simulink model "power_PVarray_grid_det"  (Simulink 8.8)
settings: Solver=FixedStepDiscrete  StartTime=0.0  StopTime=14  RelTol=1e-3
PreLoadFcn:
  | Ts_Power=1e-6;
  | Ts_Control=100e-6;
undefined symbols (not defined in the file or in its folder): D1, Delta, DiscIntNeverNeededParam, sigbuilder_block
libraries: powerlib x23, powerlib_meascontrol x11, simulink x2, re_lib x1
(part 1 of 2)
Description:
  | Copyright 2008-2016 The MathWorks, Inc.
settings Model: SuppressorTable=22 serialization::archive 11 0 3 0 0 0 11 0  Creator=MathWorks  LastModifiedBy=oka  SimulationMode=accelerator
settings DataIOCC: SignalLogging=off  DSMLogging=off
settings OptimizationCC: ExpressionDepthLimit=2147483647
settings DebuggingCC: SolverPrmCheckMsg=warning
settings ConfigComp: CovSFcnEnable=off

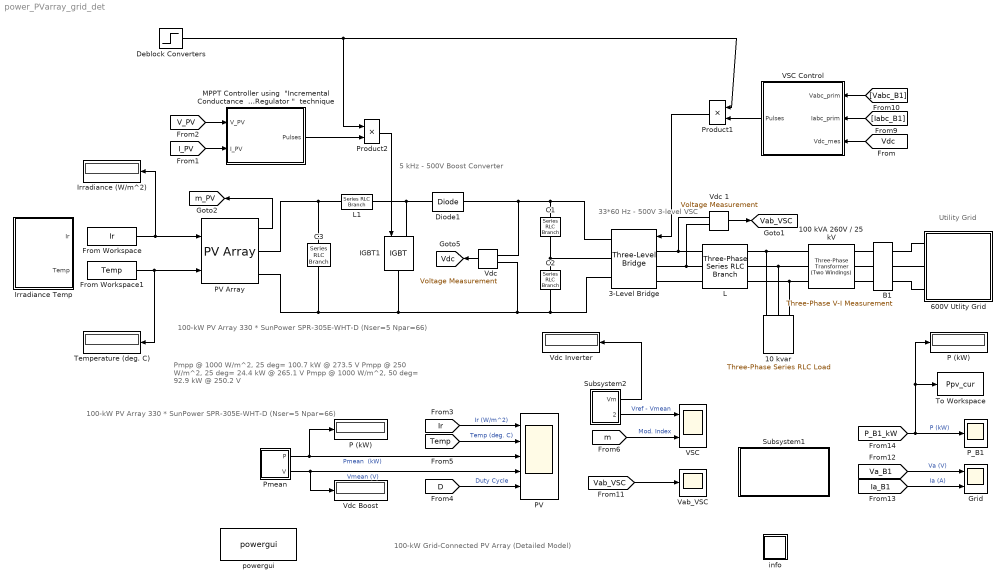
== system power_PVarray_grid_det ==
  note: 5 kHz - 500V
      | Boost Converter
  note: 33*60 Hz - 500V
      | 3-level VSC
  note: 100-kW Grid-Connected PV Array (Detailed Model)
  note: Utility Grid
  note: Pmpp @ 1000 W/m^2, 25 deg= 100.7 kW @ 273.5 V
      | Pmpp @  250 W/m^2, 25 deg= 24.4  kW @ 265.1 V
      | Pmpp @ 1000 W/m^2, 50 deg= 92.9  kW @ 250.2 V
  note: 100-kW  PV Array
      | 330 * SunPower SPR-305E-WHT-D  (Nser=5 Npar=66)
  note: 100-kW  PV Array
      | 330 * SunPower SPR-305E-WHT-D  (Nser=5 Npar=66)
  10 kvar : powerlib/Elements/Three-Phase Series RLC Load  LConnTagsString=A|B|C  Configuration=Y (grounded)  NominalVoltage=240  Vabc=[1e3 1e3 1e3]  Vabcp=[1e3 1e3 1e3]  NominalFrequency=60  UnbalancedPower=off  ActivePower=10e3/100  InductivePower=0  CapacitivePower=10e3  Pabc=[10e3 9e3 11e3]  QLabc=[100 90 110]  QCabc=[100 90 110]  Pabcp=[10e3 9e3 11e3]  QLabcp=[100 90 110]  QCabcp=[100 90 110]  Measurements=None  LoadType=constant Z
  100 kVA 260V / 25 kV : powerlib/Elements/Three-Phase Transformer (Two Windings)  Winding1Connection=Yg  Winding2Connection=Delta (D1)  CoreType=Three single-phase transformers  SetSaturation=off  Hysteresis=off  DataFile='hysteresis'  SetInitialFlux=off  Measurements=None  UNITS=pu  NominalPower=[100e3 , 60 ]  Winding1=[ 25e3 , 0.001 , 0.03 ]  Winding2=[ 260 , 0.001 , 0.03 ]  Rm=500  Lm=500  L0=0.5  Saturation=[ 0,0 ; 0.0024,1.2 ; 1.0,1.52 ]  InitialFluxes=[ 0.8 , -0.8 , 0.7 ]  MoreParameters=off  BreakLoop=off  DataType=off  TransfoNumber=0
  3-Level Bridge : powerlib/Power Electronics/Three-Level Bridge  Arms=3  SnubberResistance=1e6  SbubberCapacitance=inf  Device=IGBT / Diodes  Ron=0.2e-3  ForwardVoltages="[  0  0 ]"  Measurements=None
  600V Utlity Grid : Subsystem
      mask Display: image(imread('grid.jpg'))
  B1 : powerlib/Measurements/Three-Phase V-I Measurement  VoltageMeasurement=phase-to-ground  SetLabelV=on  LabelV=Vabc_B1  Vpu=off  VpuLL=off  CurrentMeasurement=yes  SetLabelI=on  LabelI=Iabc_B1  Ipu=off  Pbase=100e6  Vbase=500e3  OutputType=Magnitude  PhasorSimulation=off  PSBequivalent=0
  C1 : powerlib/Elements/Series RLC Branch  LConnTagsString=__new0  RConnTagsString=__new0  BranchType=C  Resistance=1.0  Inductance=1.0  SetiL0=off  InitialCurrent=0  Capacitance=12000e-06  Setx0=off  InitialVoltage=0  Measurements=None
  C2 : powerlib/Elements/Series RLC Branch  LConnTagsString=__new0  RConnTagsString=__new0  BranchType=C  Resistance=1.0  Inductance=1.0  SetiL0=off  InitialCurrent=0  Capacitance=12000e-06  Setx0=off  InitialVoltage=0  Measurements=None
  C3 : powerlib/Elements/Series RLC Branch  LConnTagsString=__new0  RConnTagsString=__new0  BranchType=C  Resistance=1.0  Inductance=1.0  SetiL0=off  InitialCurrent=0  Capacitance=100e-6  Setx0=off  InitialVoltage=0  Measurements=Branch voltage
  Deblock Converters : Step  Time=0.05  SampleTime=0
  Diode1 : powerlib/Power Electronics/Diode  Ron=1e-4  Lon=0  Vf=0  IC=0  UseSnubber=off  Rs=inf  Cs=inf  Measurements=off
  From Workspace : FromWorkspace  VariableName=Ir  SampleTime=0
  From Workspace1 : FromWorkspace  VariableName=Temp  SampleTime=0
  Grid : Scope  NumInputPorts=2
  IGBT1 : powerlib/Power Electronics/IGBT  Ron=0.001  Lon=0  Vf=0  Tf=0  Tt=0  IC=0  Rs=1e5  Cs=inf  Measurements=off
  Irradiance (W/m^2) : Display
      settings: Format=bank  Decimation=1000
  Irradiance Temp : Subsystem  Tag=STV Subsys  LoadFcn=sigbuilder_block('load');  StartFcn=sigbuilder_block('start');  StopFcn=sigbuilder_block('stop');  ClipboardFcn=sigbuilder_block('clipboard');  mask(Sigbuilder block){tuvar=[0:10]}
      mask help: Sigbuilder GUI
      mask init:
      | if ~strcmp(get_param(bdroot(gcbh),'SimulationStatus'),'stopped') tuvar = sigbuilder_block('maskInit'); end
      settings: CopyFcn=sigbuilder_block('copy');  DeleteFcn=sigbuilder_block('delete');  ModelCloseFcn=sigbuilder_block('modelClose');  PreSaveFcn=sigbuilder_block('preSave');  PauseFcn=sigbuilder_block('pause')  ContinueFcn=sigbuilder_block('continue')  NameChangeFcn=sigbuilder_block('namechange');  OpenFcn=sigbuilder_block('open',[281.25 84 564.75 395.25 ]);  CloseFcn=sigbuilder_block('close');
      mask Display: plot(0,0,100,100,[10,10,40,40,10],[80,20,20,80,80],[40,10],[50,50], [40,27,10],[65,72,56],[40,25,25,10],[28,28,43,43]);
  L : powerlib/Elements/Three-Phase Series RLC Branch  LConnTagsString=A|B|C  RConnTagsString=A|B|C  BranchType=RL  Resistance=500e-6*377/50/2  Inductance=500e-6/2  Capacitance=inf  Measurements=None
  L1 : powerlib/Elements/Series RLC Branch  LConnTagsString=__new0  RConnTagsString=__new0  BranchType=RL  Resistance=0.005  Inductance=5e-3  SetiL0=off  InitialCurrent=0  Capacitance=1e-6  Setx0=off  InitialVoltage=0  Measurements=None
  "MPPT Controller using  \"Incremental Conductance  + Integral Regulator \"  technique " : Subsystem  mask(Boost Control - MPPT){fc=5000, T_MPPT=200e-6, Dinit=0.5}
      mask prompts: fc "PWM switching frequency (Hz)"; T_MPPT "Time window used by MPPT control (s)"; Dinit "Initial value of duty cycle"
  P (kW) : Display
      settings: Format=bank  Decimation=2000
  "P (kW) " : Display
      settings: Format=bank  Decimation=2000
  PV : Scope  NumInputPorts=5
  PV Array : re_lib/Solar/PV Array  Npar=66  Nser=5  PlotType=array @ 1000 W/m2 & specified temperatures  S_vec="[ 1000  250 ]"  Temp_C_vec="[0 25 50  ]"  ModuleName=SunPower SPR-305E-WHT-D  PlotWhenSelected=off  Pm=305.226  Ncell=96  Voc=64.2  Isc=5.96  Vm=54.7  Im=5.58  beta_Voc_pc=-0.27269  alpha_Isc_pc=0.061745  beta_Voc=-0.17507  alpha_Isc=0.00368  IL=6.0092  I0=6.3014e-12  nI=0.94504  Rsh=269.5934  Rs=0.37152  BAL=on  Tc=Tc  Tfilter=5e-5
  P_B1 : Scope
  Pmean : Subsystem
  Product1 : Product  RndMeth=Zero
  Product2 : Product  RndMeth=Zero
  Subsystem1 : Subsystem
      mask Display: disp('Open this block\nto display additional \nscopes & measurements')
  Subsystem2 : Subsystem
  Temperature (deg. C) : Display
      settings: Format=bank  Decimation=1000
  To Workspace : ToWorkspace  VariableName=Ppv_cur  SaveFormat=Structure  SampleTime=-1
  VSC : Scope  NumInputPorts=2
  VSC Control : Subsystem  mask(VSC Main Controller){nom=[ 100e3  60 ], Vnom=[ 25e3 260 ], Vnom_dc=500, RLxfo=[0.002  0.06 ], RLchoke=[2e-3  250e-6  ], K_VDCreg=[7  800], K_Ireg=[0.3 20], Ts=Ts_Control}
      mask prompts: nom "Nominal power and frequency [ Pnom(VA)  Fnom(Hz) ]:"; Vnom "Nominal primary and secondary voltages (Vrms LL) [ Vnom_prim   Vnom_sec ]:"; Vnom_dc "Nominal DC bus voltage (V):"; RLxfo "Total transformer leakage impedance (pu/Pnom) [ Rxfo  Lxf ]"; RLchoke "Choke impedance [ R(ohm) L(H) ]"; K_VDCreg "VDC regultator gains [ Kp  Ki ]:"; K_Ireg "Current regulator gains [ Kp  Ki ]:"; Ts "Sample time"
      mask init:
      | Pnom=nom(1);
      | Fnom=nom(2);
      | Vnom_prim=Vnom(1);
      | Vnom_sec=Vnom(2);
      | Zbase=Vnom_sec^2/Pnom;
      | Rtot_pu=RLxfo(1) + RLchoke(1)/Zbase;
      | Ltot_pu=RLxfo(2) + RLchoke(2)/(Zbase/(2*pi*Fnom));
      | Kp_VDCreg=K_VDCreg(1);
      | Ki_VDCreg=K_VDCreg(2);
      | Kp_Ireg=K_Ireg(1);
      | Ki_Ireg=K_Ireg(2);
      | Vdc_ref=Vnom_dc;
      | % Used to determine initial value of Boost Control (MPPT)
      | assignin('base','Vdc_ref_Inv',Vdc_ref);
  Vab_VSC : Scope
  "Vdc " : powerlib/Measurements/Voltage Measurement  Tag=PoWeRsYsTeMmEaSuReMeNt  PhasorSimulation=off  OutputType=Magnitude  PSBequivalent=0
  Vdc 1 : powerlib/Measurements/Voltage Measurement  Tag=PoWeRsYsTeMmEaSuReMeNt  PhasorSimulation=off  OutputType=Magnitude  PSBequivalent=0
  Vdc Boost : Display
      settings: Format=bank  Decimation=2000
  Vdc Inverter : Display
      settings: Format=bank  Decimation=2000
  info : Subsystem
      settings: OpenFcn=showdemo(bdroot(gcb))
      mask Display: disp('?')
  powergui : powerlib/powergui  Priority=1  SimulationMode=Discrete  SolverType=Tustin/Backward Euler (TBE)  SampleTime=Ts_Power  frequency=60  SPID=off  DisableSnubberDevices=off  DisableRonSwitches=off  DisableVfSwitches=off  SwTol=0  DisplayEquations=off  Interpol=off  ExternalGateDelay=off  methode=off  Ts=0  FunctionMessages=off  echomessages=off  HookPort=off  EnableUseOfTLC=off  x0status=blocks  frequencyindice=0  Pbase=100e6  ErrMax=1e-4  Iterations=50  UnitsV=kV  UnitsW=MW  buscounter=0  RestoreLinks=warning  ResistiveCurrentMeasurement=off  Frange=[0:2:500]  Ylog=off  Xlog=on  ShowGrid=off  save=off  variable=ZData  structure=0  ZoomFFT=on  StartTime=0.0  cycles=1  DisplayStyle=1  fundamental=60  FreqAxis=off  MaxFrequency=1000  frequencyindicesteady=1  RmsSteady=1  display=off
  tag scope: Vab_VSC=global, Vdc=global, m_PV=global
  wires:
  "Vdc "/1 -> [Vdc]
  Product2/1 -> IGBT1/1
  "MPPT Controller using  \"Incremental Conductance  + Integral Regulator \"  technique "/1(Pulses) -> Product2/2
  Deblock Converters/1 -> Product2/1, Product1/1
  [Vabc_B1] -> VSC Control/1(Vabc_prim)
  [Iabc_B1] -> VSC Control/2(Iabc_prim)
  [Vdc] -> VSC Control/3(Vdc_mes)
  VSC Control/1(Pulses) -> Product1/2
  Product1/1 -> 3-Level Bridge/1
  [I_PV] -> "MPPT Controller using  \"Incremental Conductance  + Integral Regulator \"  technique "/2(I_PV)
  [V_PV] -> "MPPT Controller using  \"Incremental Conductance  + Integral Regulator \"  technique "/1(V_PV)
  Pmean/1(P) -> "P (kW) "/1, PV/3  "Pmean  (kW)"
  [m] -> VSC/2  "Mod. Index"
  Vdc 1/1 -> [Vab_VSC]
  [Vab_VSC] -> Vab_VSC/1
  [Ia_B1] -> Grid/2  "Ia (A)"
  [Va_B1] -> Grid/1  "Va (V)"
  [P_B1_kW] -> P_B1/1, To Workspace/1, P (kW)/1  "P (kW)"
  Pmean/2(V) -> Vdc Boost/1, PV/4  "Vmean (V)"
  Subsystem2/2(VrVm) -> VSC/1  "Vref - Vmean"
  Subsystem2/1(Vm) -> Vdc Inverter/1
  PV Array/1 -> [m_PV]
  From Workspace/1 -> PV Array/1, Irradiance (W/m^2)/1
  From Workspace1/1 -> PV Array/2, Temperature (deg. C)/1
  [D] -> PV/5  "Duty Cycle"
  [Temp] -> PV/2  "Temp (deg. C)"
  [Ir] -> PV/1  "Ir (W/m^2)"
  connections:
  3-Level Bridge/RConn1 -- Diode1/RConn1 -- "Vdc "/LConn1 -- C1/LConn1
  L1/RConn1 -- Diode1/LConn1 -- IGBT1/LConn1
  3-Level Bridge/RConn3 -- C2/RConn1 -- "Vdc "/LConn2 -- IGBT1/RConn1 -- PV Array/RConn2 -- C3/RConn1
  3-Level Bridge/LConn1 -- L/LConn1 -- Vdc 1/LConn1
  3-Level Bridge/LConn2 -- L/LConn2 -- Vdc 1/LConn2
  3-Level Bridge/LConn3 -- L/LConn3
  L/RConn1 -- 100 kVA 260V / 25 kV/RConn1 -- 10 kvar/LConn1
  L/RConn2 -- 100 kVA 260V / 25 kV/RConn2 -- 10 kvar/LConn2
  L/RConn3 -- 100 kVA 260V / 25 kV/RConn3 -- 10 kvar/LConn3
  B1/LConn1 -- 100 kVA 260V / 25 kV/LConn1
  B1/LConn2 -- 100 kVA 260V / 25 kV/LConn2
  B1/LConn3 -- 100 kVA 260V / 25 kV/LConn3
  C2/LConn1 -- C1/RConn1 -- 3-Level Bridge/RConn2
  C3/LConn1 -- PV Array/RConn1 -- L1/LConn1
  B1/RConn2 -- 600V Utlity Grid/LConn2
  B1/RConn1 -- 600V Utlity Grid/LConn1
  B1/RConn3 -- 600V Utlity Grid/LConn3

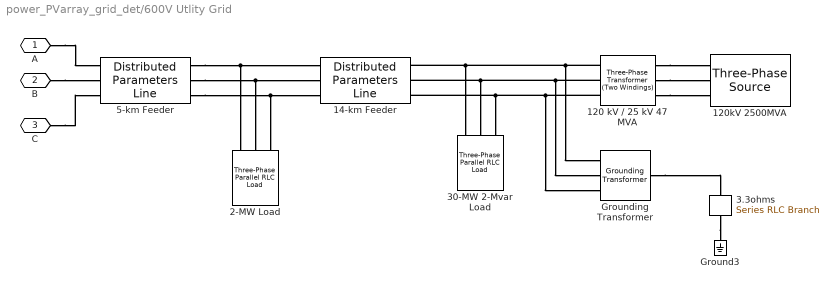
== system power_PVarray_grid_det/600V Utlity Grid ==
  120 kV / 25 kV 47 MVA : powerlib/Elements/Three-Phase Transformer (Two Windings)  Winding1Connection=Yg  Winding2Connection=Delta (D1)  CoreType=Three single-phase transformers  SetSaturation=off  Hysteresis=off  DataFile='basic_model'  SetInitialFlux=off  Measurements=None  UNITS=pu  NominalPower=[47e6 60 ]  Winding1="[ 120e3  0.08/30   0.08 ]"  Winding2="[ 25e3  0.08/30  0.08]"  Rm=500  Lm=500  L0=0.5  Saturation="[ 0,0  ;  0.005,1.2  ;  1.0,1.4 ]"  InitialFluxes=[ 0.8 , -0.8 , 0.7 ]  MoreParameters=off  BreakLoop=off  DataType=off  TransfoNumber=0
  120kV 2500MVA : powerlib/Electrical Sources/Three-Phase Source  InternalConnection=Yg  VoltagePhases=off  Voltage=120e3  PhaseAngle=0  Voltage_phases=[25e3 25e3 25e3]/sqrt(3)  PhaseAngles_phases=[0 -120 +120]  Frequency=60  NonIdealSource=on  SpecifyImpedance=on  Resistance=0.8929  Inductance=16.58e-3  ShortCircuitLevel=2500e6  BaseVoltage=120e3  XRratio=7  BusType=swing  Pref=0  Qref=0  Prefabc=[10e3, 10e3, 10e3]  Qrefabc=[0, 0, 0]  Qmin=-inf  Qmax=inf
  14-km Feeder : powerlib/Elements/Distributed Parameters Line  Phases=3  Frequency=60  Resistance=[0.1153 0.413]  Inductance=[1.05e-3 3.32e-3]  Capacitance=[11.33e-009 5.01e-009]  Length=14  x1=[-5.8e-05 -2.28725950777772e-09 0 0;-5.7e-05 -2.28813335663527e-09 0 0;-5.6e-05 -2.28900688029804e-09 0 0;-5.5e-05 -2.28988007864189e-09 0 0;-5.4e-05 -2.2907529515427e-09 0 0;-5.3e-05 -2.29162549887644e-09 0 0;-5.2e-05 -2.29249772051908e-09 0 0;-5.1e-05 -2.29336961634667e-09 0 0;-5e-05 -2.29424118623529e-09 0 0;-4.9e-05 -2.29511243006108e-09 -3790.73535189758 -24061.4134200285;-4.8e-05 -2.2959833477002e-09 -3781.66414358219 -24062.8407837229;-4.7e-05 -2.29685393902889e-09 -3772.59239780798 -24064.264727551;-4.6e-05 -2.2977242039234e-09 -3763.52011586426 -24065.6852513104;-4.5e-05 -2.29859414226007e-09 -3754.4472990404 -24067.1023547992;-4.4e-05 -2.29946375391524e-09 -3745.37394862584 -24068.516037816;-4.3e-05 -2.30033303876533e-09 -3736.30006591012 -24069.92630016;-4.2e-05 -2.3012019966868e-09 -3727.22565218283 -24071.3331416306;-4.1e-05 -2.30207062755614e-09 -3718.15070873366 -24072.7365620279;-4e-05 -2.30293893124991e-09 -3709.07523685234 -24074.1365611525;-3.9e-05 -2.30380690764469e-09 -3699.99923782872 -24075.5331388054;-3.8e-05 -2.30467455661714e-09 -3690.92271295269 -24076.9262947882;-3.7e-05 -2.30554187804393e-09 -3681.84566351423 -24078.3160289027;-3.6e-05 -2.3064088718018e-09 -3672.76809080339 -24079.7023409516;-3.5e-05 -2.30727553776754e-09 -3663.68999611029 -24081.0852307377;-3.4e-05 -2.30814187581796e-09 -3654.61138072514 -24082.4646980646;-3.3e-05 -2.30900788582995e-09 -3645.53224593821 -24083.8407427361;-3.2e-05 -2.30987356768043e-09 -3636.45259303984 -24085.2133645568;-3.1e-05 -2.31073892124635e-09 -3627.37242332047 -24086.5825633315;-3e-05 -2.31160394640474e-09 -3618.29173807057 -24087.9483388657;-2.9e-05 -2.31246864303266e-09 -3609.21053858072 -24089.3106909652;-2.8e-05 -2.31333301100722e-09 -3600.12882614157 -24090.6696194364;-2.7e-05 -2.31419705020556e-09 -3591.04660204382 -24092.0251240862;-2.6e-05 -2.31506076050488e-09 -3581.96386757826 -24093.377204722;-2.5e-05 -2.31592414178245e-09 -3572.88062403575 -24094.7258611515;-2.4e-05 -2.31678719391554e-09 -3563.79687270722 -24096.0710931831;-2.3e-05 -2.31764991678151e-09 -3554.71261488368 -24097.4129006256;-2.2e-05 -2.31851231025774e-09 -3545.6278518562 -24098.7512832884;-2.1e-05 -2.31937437422166e-09 -3536.54258491593 -24100.0862409811;-2e-05 -2.32023610855075e-09 -3527.45681535409 -24101.4177735141;-1.9e-05 -2.32109751312255e-09 -3518.37054446196 -24102.7458806982;-1.8e-05 -2.32195858781463e-09 -3509.28377353092 -24104.0705623445;-1.7e-05 -2.32281933250461e-09 -3500.19650385239 -24105.3918182649;-1.6e-05 -2.32367974707016e-09 -3491.10873671787 -24106.7096482714;-1.5e-05 -2.324539831389e-09 -3482.02047341895 -24108.024052177;-1.4e-05 -2.32539958533888e-09 -3472.93171524726 -24109.3350297946;-1.3e-05 -2.32625900879762e-09 -3463.84246349452 -24110.6425809381;-1.2e-05 -2.32711810164308e-09 -3454.75271945252 -24111.9467054215;-1.1e-05 -2.32797686375316e-09 -3445.66248441311 -24113.2474030596;-1e-05 -2.3288352950058e-09 -3436.57175966822 -24114.5446736674;-9e-06 -2.32969339527902e-09 -3427.48054650984 -24115.8385170607;-8e-06 -2.33055116445085e-09 -3418.38884623003 -24117.1289330555;-7e-06 -2.33140860239938e-09 -3409.29666012093 -24118.4159214684;-6e-06 -2.33226570900275e-09 -3400.20398947475 -24119.6994821165;-5e-06 -2.33312248413916e-09 -3391.11083558375 -24120.9796148174;-4e-06 -2.33397892768682e-09 -3382.01719974027 -24122.2563193892;-3e-06 -2.33483503952403e-09 -3372.92308323672 -24123.5295956504;-2e-06 -2.33569081952911e-09 -3363.82848736558 -24124.79944342;-1e-06 -2.33654626758044e-09 -3354.73341341939 -24126.0658625176]  x2=[-5.8e-05 -2.52305968273904e-09 0 0;-5.7e-05 -2.52396169480787e-09 0 0;-5.6e-05 -2.52486334816545e-09 0 0;-5.5e-05 -2.52576464268364e-09 0 0;-5.4e-05 -2.52666557823435e-09 0 0;-5.3e-05 -2.52756615468953e-09 0 0;-5.2e-05 -2.52846637192119e-09 0 0;-5.1e-05 -2.52936622980139e-09 0 0;-5e-05 -2.53026572820224e-09 0 0;-4.9e-05 -2.5311648669959e-09 -3379.39242591105 -24244.0512732186;-4.8e-05 -2.53206364605458e-09 -3370.25239397924 -24245.3235513085;-4.7e-05 -2.53296206525055e-09 -3361.11188305941 -24246.5923835972;-4.6e-05 -2.53386012445612e-09 -3351.97089445062 -24247.8577699044;-4.5e-05 -2.53475782354366e-09 -3342.82942945201 -24249.1197100502;-4.4e-05 -2.53565516238559e-09 -3333.68748936279 -24250.3782038553;-4.3e-05 -2.53655214085436e-09 -3324.54507548223 -24251.6332511409;-4.2e-05 -2.5374487588225e-09 -3315.40218910968 -24252.8848517285;-4.1e-05 -2.53834501616259e-09 -3306.25883154453 -24254.1330054403;-4e-05 -2.53924091274724e-09 -3297.11500408626 -24255.3777120989;-3.9e-05 -2.54013644844913e-09 -3287.97070803443 -24256.6189715274;-3.8e-05 -2.54103162314098e-09 -3278.82594468863 -24257.8567835494;-3.7e-05 -2.54192643669557e-09 -3269.68071534854 -24259.0911479889;-3.6e-05 -2.54282088898572e-09 -3260.5350213139 -24260.3220646705;-3.5e-05 -2.54371497988431e-09 -3251.38886388451 -24261.5495334194;-3.4e-05 -2.54460870926428e-09 -3242.24224436026 -24262.773554061;-3.3e-05 -2.54550207699859e-09 -3233.09516404108 -24263.9941264213;-3.2e-05 -2.5463950829603e-09 -3223.94762422697 -24265.211250327;-3.1e-05 -2.54728772702247e-09 -3214.79962621801 -24266.424925605;-3e-05 -2.54818000905825e-09 -3205.65117131432 -24267.6351520828;-2.9e-05 -2.54907192894082e-09 -3196.50226081611 -24268.8419295885;-2.8e-05 -2.54996348654342e-09 -3187.35289602364 -24270.0452579505;-2.7e-05 -2.55085468173935e-09 -3178.20307823724 -24271.2451369978;-2.6e-05 -2.55174551440193e-09 -3169.05280875731 -24272.4415665598;-2.5e-05 -2.55263598440457e-09 -3159.90208888429 -24273.6345464666;-2.4e-05 -2.5535260916207e-09 -3150.75091991872 -24274.8240765486;-2.3e-05 -2.55441583592383e-09 -3141.59930316117 -24276.0101566368;-2.2e-05 -2.5553052171875e-09 -3132.4472399123 -24277.1927865624;-2.1e-05 -2.55619423528532e-09 -3123.29473147282 -24278.3719661576;-2e-05 -2.55708289009092e-09 -3114.1417791435 -24279.5476952547;-1.9e-05 -2.55797118147802e-09 -3104.98838422519 -24280.7199736865;-1.8e-05 -2.55885910932037e-09 -3095.83454801878 -24281.8888012866;-1.7e-05 -2.55974667349177e-09 -3086.68027182524 -24283.0541778887;-1.6e-05 -2.56063387386608e-09 -3077.52555694559 -24284.2161033273;-1.5e-05 -2.56152071031721e-09 -3068.37040468093 -24285.3745774372;-1.4e-05 -2.56240718271912e-09 -3059.2148163324 -24286.5296000537;-1.3e-05 -2.56329329094583e-09 -3050.05879320122 -24287.6811710128;-1.2e-05 -2.56417903487139e-09 -3040.90233658867 -24288.8292901507;-1.1e-05 -2.56506441436993e-09 -3031.74544779607 -24289.9739573043;-1e-05 -2.56594942931561e-09 -3022.58812812484 -24291.1151723109;-9e-06 -2.56683407958265e-09 -3013.43037887642 -24292.2529350083;-8e-06 -2.56771836504532e-09 -3004.27220135234 -24293.3872452348;-7e-06 -2.56860228557795e-09 -2995.11359685418 -24294.5181028291;-6e-06 -2.56948584105491e-09 -2985.95456668359 -24295.6455076307;-5e-06 -2.57036903135062e-09 -2976.79511214226 -24296.7694594792;-4e-06 -2.57125185633958e-09 -2967.63523453195 -24297.8899582148;-3e-06 -2.5721343158963e-09 -2958.4749351545 -24299.0070036785;-2e-06 -2.57301640989537e-09 -2949.31421531177 -24300.1205957113;-1e-06 -2.57389813821143e-09 -2940.15307630573 -24301.2307341551]  x3=[-5.8e-05 -3.16003121714594e-12 0 0;-5.7e-05 -3.16595959451391e-12 0 0;-5.6e-05 -3.17188752192842e-12 0 0;-5.5e-05 -3.17781499854697e-12 0 0;-5.4e-05 -3.18374202352714e-12 0 0;-5.3e-05 -3.18966859602657e-12 0 0;-5.2e-05 -3.19559471520295e-12 0 0;-5.1e-05 -3.20152038021406e-12 0 0;-5e-05 -3.20744559021773e-12 0 0;-4.9e-05 -3.21337034437184e-12 -23.5442847382511 -155.681477773845;-4.8e-05 -3.21929464183436e-12 -23.4855925321324 -155.690342696966;-4.7e-05 -3.22521848176332e-12 -23.4268969881873 -155.699185493017;-4.6e-05 -3.23114186331681e-12 -23.3681981147576 -155.708006160741;-4.5e-05 -3.23706478565297e-12 -23.3094959201858 -155.716804698886;-4.4e-05 -3.24298724793004e-12 -23.2507904128148 -155.725581106199;-4.3e-05 -3.2489092493063e-12 -23.192081600988 -155.734335381435;-4.2e-05 -3.25483078894009e-12 -23.1333694930491 -155.743067523348;-4.1e-05 -3.26075186598985e-12 -23.0746540973425 -155.751777530698;-4e-05 -3.26667247961404e-12 -23.015935422213 -155.760465402247;-3.9e-05 -3.27259262897122e-12 -22.9572134760058 -155.76913113676;-3.8e-05 -3.27851231322e-12 -22.8984882670665 -155.777774733006;-3.7e-05 -3.28443153151907e-12 -22.8397598037414 -155.786396189755;-3.6e-05 -3.29035028302717e-12 -22.781028094377 -155.794995505784;-3.5e-05 -3.29626856690311e-12 -22.7222931473205 -155.803572679869;-3.4e-05 -3.30218638230578e-12 -22.6635549709194 -155.812127710792;-3.3e-05 -3.30810372839412e-12 -22.6048135735217 -155.820660597337;-3.2e-05 -3.31402060432714e-12 -22.5460689634759 -155.82917133829;-3.1e-05 -3.31993700926392e-12 -22.4873211491309 -155.837659932443;-3e-05 -3.32585294236362e-12 -22.428570138836 -155.84612637859;-2.9e-05 -3.33176840278544e-12 -22.3698159409411 -155.854570675526;-2.8e-05 -3.33768338968867e-12 -22.3110585637964 -155.862992822051;-2.7e-05 -3.34359790223265e-12 -22.2522980157528 -155.87139281697;-2.6e-05 -3.3495119395768e-12 -22.1935343051614 -155.879770659087;-2.5e-05 -3.35542550088061e-12 -22.1347674403737 -155.888126347213;-2.4e-05 -3.36133858530362e-12 -22.075997429742 -155.896459880159;-2.3e-05 -3.36725119200545e-12 -22.0172242816187 -155.904771256742;-2.2e-05 -3.37316332014579e-12 -21.9584480043569 -155.913060475779;-2.1e-05 -3.3790749688844e-12 -21.8996686063098 -155.921327536094;-2e-05 -3.3849861373811e-12 -21.8408860958315 -155.92957243651;-1.9e-05 -3.39089682479577e-12 -21.7821004812761 -155.937795175857;-1.8e-05 -3.39680703028839e-12 -21.7233117709985 -155.945995752966;-1.7e-05 -3.40271675301897e-12 -21.6645199733538 -155.95417416667;-1.6e-05 -3.40862599214761e-12 -21.6057250966977 -155.962330415809;-1.5e-05 -3.41453474683448e-12 -21.5469271493862 -155.970464499222;-1.4e-05 -3.42044301623982e-12 -21.4881261397758 -155.978576415754;-1.3e-05 -3.42635079952392e-12 -21.4293220762235 -155.986666164251;-1.2e-05 -3.43225809584715e-12 -21.3705149670866 -155.994733743564;-1.1e-05 -3.43816490436997e-12 -21.3117048207229 -156.002779152547;-1e-05 -3.44407122425288e-12 -21.2528916454906 -156.010802390056;-9e-06 -3.44997705465646e-12 -21.1940754497485 -156.01880345495;-8e-06 -3.45588239474135e-12 -21.1352562418557 -156.026782346093;-7e-06 -3.46178724366829e-12 -21.0764340301715 -156.03473906235;-6e-06 -3.46769160059806e-12 -21.017608823056 -156.042673602592;-5e-06 -3.47359546469151e-12 -20.9587806288696 -156.050585965689;-4e-06 -3.47949883510959e-12 -20.8999494559731 -156.058476150518;-3e-06 -3.48540171101328e-12 -20.8411153127276 -156.066344155957;-2e-06 -3.49130409156365e-12 -20.7822782074948 -156.074189980888;-1e-06 -3.49720597592185e-12 -20.7234381486368 -156.082013624196]  x4=[-5.8e-05 -3.06172038133671e-12 0 0;-5.7e-05 -3.05774342246562e-12 0 0;-5.6e-05 -3.053766029021e-12 0 0;-5.5e-05 -3.04978820156812e-12 0 0;-5.4e-05 -3.04580994067232e-12 0 0;-5.3e-05 -3.041831246899e-12 0 0;-5.2e-05 -3.03785212081362e-12 0 0;-5.1e-05 -3.03387256298171e-12 0 0;-5e-05 -3.02989257396885e-12 0 0;-4.9e-05 -3.02591215434068e-12 -1.35581366009316 -2.1529852269828;-4.8e-05 -3.02193130466291e-12 -1.35500190745802 -2.15349620368519;-4.7e-05 -3.01795002550131e-12 -1.3541899622469 -2.15400687432774;-4.6e-05 -3.0139683174217e-12 -1.35337782457517 -2.15451723883788;-4.5e-05 -3.00998618098998e-12 -1.35256549455828 -2.15502729714306;-4.4e-05 -3.00600361677209e-12 -1.35175297231167 -2.15553704917081;-4.3e-05 -3.00202062533406e-12 -1.35094025795081 -2.15604649484867;-4.2e-05 -2.99803720724194e-12 -1.35012735159121 -2.15655563410424;-4.1e-05 -2.99405336306187e-12 -1.34931425334841 -2.15706446686517;-4e-05 -2.99006909336005e-12 -1.34850096333795 -2.15757299305912;-3.9e-05 -2.98608439870272e-12 -1.34768748167544 -2.15808121261383;-3.8e-05 -2.98209927965621e-12 -1.34687380847648 -2.15858912545708;-3.7e-05 -2.97811373678688e-12 -1.34605994385672 -2.15909673151667;-3.6e-05 -2.97412777066118e-12 -1.34524588793182 -2.15960403072046;-3.5e-05 -2.97014138184559e-12 -1.34443164081747 -2.16011102299636;-3.4e-05 -2.96615457090667e-12 -1.34361720262941 -2.1606177082723;-3.3e-05 -2.96216733841104e-12 -1.34280257348338 -2.16112408647629;-3.2e-05 -2.95817968492536e-12 -1.34198775349515 -2.16163015753634;-3.1e-05 -2.95419161101638e-12 -1.34117274278054 -2.16213592138054;-3e-05 -2.95020311725089e-12 -1.34035754145537 -2.16264137793701;-2.9e-05 -2.94621420419574e-12 -1.3395421496355 -2.16314652713391;-2.8e-05 -2.94222487241785e-12 -1.33872656743681 -2.16365136889944;-2.7e-05 -2.93823512248419e-12 -1.33791079497523 -2.16415590316187;-2.6e-05 -2.93424495496179e-12 -1.33709483236668 -2.16466012984947;-2.5e-05 -2.93025437041774e-12 -1.33627867972714 -2.16516404889059;-2.4e-05 -2.92626336941919e-12 -1.3354623371726 -2.16566766021362;-2.3e-05 -2.92227195253337e-12 -1.33464580481907 -2.16617096374697;-2.2e-05 -2.91828012032752e-12 -1.33382908278262 -2.16667395941912;-2.1e-05 -2.91428787336899e-12 -1.3330121711793 -2.16717664715858;-2e-05 -2.91029521222515e-12 -1.33219507012522 -2.16767902689391;-1.9e-05 -2.90630213746347e-12 -1.33137777973652 -2.1681810985537;-1.8e-05 -2.90230864965143e-12 -1.33056030012934 -2.16868286206661;-1.7e-05 -2.89831474935661e-12 -1.32974263141987 -2.16918431736131;-1.6e-05 -2.89432043714662e-12 -1.32892477372431 -2.16968546436655;-1.5e-05 -2.89032571358915e-12 -1.32810672715891 -2.17018630301109;-1.4e-05 -2.88633057925194e-12 -1.32728849183992 -2.17068683322377;-1.3e-05 -2.88233503470278e-12 -1.32647006788364 -2.17118705493343;-1.2e-05 -2.87833908050954e-12 -1.32565145540638 -2.17168696806899;-1.1e-05 -2.87434271724012e-12 -1.32483265452448 -2.1721865725594;-1e-05 -2.87034594546249e-12 -1.32401366535431 -2.17268586833366;-9e-06 -2.8663487657447e-12 -1.32319448801228 -2.1731848553208;-8e-06 -2.86235117865482e-12 -1.3223751226148 -2.17368353344991;-7e-06 -2.858353184761e-12 -1.32155556927832 -2.1741819026501;-6e-06 -2.85435478463145e-12 -1.32073582811933 -2.17467996285057;-5e-06 -2.85035597883442e-12 -1.31991589925432 -2.17517771398051;-4e-06 -2.84635676793825e-12 -1.31909578279982 -2.17567515596919;-3e-06 -2.8423571525113e-12 -1.31827547887239 -2.1761722887459;-2e-06 -2.838357133122e-12 -1.31745498758862 -2.17666911224001;-1e-06 -2.83435671033886e-12 -1.31663430906511 -2.17716562638088]  x5=5.70973484498186e-05  V1=ones(3,3)  V2=ones(3,3)  I1=ones(3,3)  I2=ones(3,3)  nHarmo=1  Measurements=None
  2-MW Load : powerlib/Elements/Three-Phase Parallel RLC Load  LConnTagsString=A|B|C  Configuration=Y (grounded)  NominalVoltage=25e3  Vabc=[1e3 1e3 1e3]  Vabcp=[1e3 1e3 1e3]  NominalFrequency=60  UnbalancedPower=off  ActivePower=2e6  InductivePower=0  CapacitivePower=0  Pabc=[10e3 9e3 11e3]  QLabc=[100 90 110]  QCabc=[100 90 110]  Pabcp=[10e3 9e3 11e3]  QLabcp=[100 90 110]  QCabcp=[100 90 110]  Measurements=None  LoadType=constant Z
  "3.3ohms " : powerlib/Elements/Series RLC Branch  LConnTagsString=__new0  RConnTagsString=__new0  BranchType=R  Resistance=3.3  Inductance=[]  SetiL0=off  InitialCurrent=0  Capacitance=[]  Setx0=off  InitialVoltage=0  Measurements=None
  30-MW 2-Mvar Load : powerlib/Elements/Three-Phase Parallel RLC Load  LConnTagsString=A|B|C  Configuration=Y (grounded)  NominalVoltage=25e3  Vabc=[1e3 1e3 1e3]  Vabcp=[1e3 1e3 1e3]  NominalFrequency=60  UnbalancedPower=off  ActivePower=30e6  InductivePower=2e6  CapacitivePower=0  Pabc=[10e3 9e3 11e3]  QLabc=[100 90 110]  QCabc=[100 90 110]  Pabcp=[10e3 9e3 11e3]  QLabcp=[100 90 110]  QCabcp=[100 90 110]  Measurements=None  LoadType=constant Z
  5-km Feeder : powerlib/Elements/Distributed Parameters Line  Phases=3  Frequency=60  Resistance=[0.1153 0.413]  Inductance=[1.05e-3 3.32e-3]  Capacitance=[11.33e-009 5.01e-009]  Length=5  x1=[-2.1e-05 -2.29057926542131e-09 -3537.17773129417 -24101.4118174724;-2e-05 -2.29142625764143e-09 -3528.09146195665 -24102.7435893557;-1.9e-05 -2.29227292419878e-09 -3519.00469119864 -24104.0719357017;-1.8e-05 -2.29311926497303e-09 -3509.91742031158 -24105.3968563215;-1.7e-05 -2.29396527984388e-09 -3500.82965058698 -24106.7183510268;-1.6e-05 -2.29481096869112e-09 -3491.74138331642 -24108.0364196298;-1.5e-05 -2.29565633139453e-09 -3482.65261979153 -24109.3510619432;-1.4e-05 -2.29650136783399e-09 -3473.56336130404 -24110.6622777801;-1.3e-05 -2.29734607788938e-09 -3464.47360914572 -24111.9700669541;-1.2e-05 -2.29819046144066e-09 -3455.38336460845 -24113.2744292796;-1.1e-05 -2.29903451836783e-09 -3446.29262898413 -24114.5753645709;-1e-05 -2.29987824855091e-09 -3437.20140356478 -24115.8728726433;-9e-06 -2.30072165187001e-09 -3428.10968964245 -24117.1669533123;-8e-06 -2.30156472820525e-09 -3419.01748850928 -24118.4576063941;-7e-06 -2.30240747743681e-09 -3409.92480145747 -24119.7448317051;-6e-06 -2.30324989944492e-09 -3400.83162977931 -24121.0286290625;-5e-06 -2.30409199410986e-09 -3391.73797476712 -24122.3089982838;-4e-06 -2.30493376131194e-09 -3382.64383771333 -24123.585939187;-3e-06 -2.30577520093152e-09 -3373.54921991041 -24124.8594515906;-2e-06 -2.30661631284903e-09 -3364.45412265091 -24126.1295353137;-1e-06 -2.30745709694492e-09 -3355.35854722744 -24127.3961901757]  x2=[-2.1e-05 -2.3184613079091e-09 -3536.54258491593 -24100.0862409811;-2e-05 -2.31932321101899e-09 -3527.45681535409 -24101.4177735141;-1.9e-05 -2.32018478450133e-09 -3518.37054446196 -24102.7458806982;-1.8e-05 -2.32104602823367e-09 -3509.28377353092 -24104.0705623445;-1.7e-05 -2.32190694209361e-09 -3500.19650385239 -24105.3918182649;-1.6e-05 -2.32276752595879e-09 -3491.10873671787 -24106.7096482714;-1.5e-05 -2.32362777970689e-09 -3482.02047341895 -24108.024052177;-1.4e-05 -2.32448770321568e-09 -3472.93171524726 -24109.3350297946;-1.3e-05 -2.32534729636291e-09 -3463.84246349452 -24110.6425809381;-1.2e-05 -2.32620655902644e-09 -3454.75271945252 -24111.9467054215;-1.1e-05 -2.32706549108414e-09 -3445.66248441311 -24113.2474030596;-1e-05 -2.32792409241394e-09 -3436.57175966822 -24114.5446736674;-9e-06 -2.3287823628938e-09 -3427.48054650984 -24115.8385170607;-8e-06 -2.32964030240175e-09 -3418.38884623003 -24117.1289330555;-7e-06 -2.33049791081587e-09 -3409.29666012093 -24118.4159214684;-6e-06 -2.33135518801425e-09 -3400.20398947475 -24119.6994821165;-5e-06 -2.33221213387507e-09 -3391.11083558375 -24120.9796148174;-4e-06 -2.33306874827654e-09 -3382.01719974027 -24122.2563193892;-3e-06 -2.3339250310969e-09 -3372.92308323672 -24123.5295956504;-2e-06 -2.33478098221446e-09 -3363.82848736558 -24124.79944342;-1e-06 -2.33563660150758e-09 -3354.73341341939 -24126.0658625176]  x3=[-2.1e-05 6.08370531311982e-13 -11.1569792961284 -79.1361755515124;-2e-05 6.04746622608427e-13 -11.1271448686778 -79.1403760100082;-1.9e-05 6.0112262795689e-13 -11.0973088598117 -79.1445652208916;-1.8e-05 5.97498547872422e-13 -11.0674712737706 -79.1487431835672;-1.7e-05 5.93874382870085e-13 -11.037632114795 -79.1529098974413;-1.6e-05 5.90250133464953e-13 -11.0077913871257 -79.1570653619217;-1.5e-05 5.86625800172114e-13 -10.9779490950037 -79.1612095764177;-1.4e-05 5.83001383506666e-13 -10.9481052426703 -79.1653425403404;-1.3e-05 5.7937688398372e-13 -10.9182598343671 -79.1694642531024;-1.2e-05 5.75752302118397e-13 -10.8884128743356 -79.173574714118;-1.1e-05 5.72127638425832e-13 -10.8585643668178 -79.1776739228028;-1e-05 5.6850289342117e-13 -10.8287143160559 -79.1817618785744;-9e-06 5.64878067619568e-13 -10.7988627262921 -79.1858385808518;-8e-06 5.61253161536195e-13 -10.7690096017692 -79.1899040290555;-7e-06 5.57628175686231e-13 -10.7391549467297 -79.1939582226078;-6e-06 5.54003110584867e-13 -10.7092987654169 -79.1980011609324;-5e-06 5.50377966747306e-13 -10.6794410620739 -79.2020328434549;-4e-06 5.46752744688761e-13 -10.6495818409442 -79.2060532696021;-3e-06 5.43127444924458e-13 -10.6197211062713 -79.2100624388027;-2e-06 5.39502067969633e-13 -10.5898588622993 -79.214060350487;-1e-06 5.35876614339531e-13 -10.5599951132721 -79.2180470040867]  x4=[-2.1e-05 -8.83317216456351e-12 -12.5606324025968 -78.9000787577191;-2e-05 -8.83207682575684e-12 -12.5308868817932 -78.9048083977342;-1.9e-05 -8.83098023171508e-12 -12.5011395800712 -78.9095268236163;-1.8e-05 -8.82988238259409e-12 -12.4713905016584 -78.9142340346948;-1.7e-05 -8.8287832785499e-12 -12.4416396507828 -78.9189300303008;-1.6e-05 -8.8276829197387e-12 -12.4118870316728 -78.9236148097667;-1.5e-05 -8.82658130631688e-12 -12.3821326485569 -78.9282883724269;-1.4e-05 -8.82547843844102e-12 -12.3523765056638 -78.9329507176171;-1.3e-05 -8.82437431626784e-12 -12.3226186072225 -78.9376018446746;-1.2e-05 -8.82326893995428e-12 -12.2928589574622 -78.9422417529385;-1.1e-05 -8.82216230965742e-12 -12.2630975606126 -78.9468704417492;-1e-05 -8.82105442553455e-12 -12.2333344209033 -78.951487910449;-9e-06 -8.81994528774313e-12 -12.2035695425644 -78.9560941583817;-8e-06 -8.81883489644078e-12 -12.173802929826 -78.9606891848925;-7e-06 -8.81772325178532e-12 -12.1440345869188 -78.9652729893284;-6e-06 -8.81661035393473e-12 -12.1142645180734 -78.969845571038;-5e-06 -8.81549620304718e-12 -12.0844927275209 -78.9744069293713;-4e-06 -8.81438079928102e-12 -12.0547192194925 -78.9789570636801;-3e-06 -8.81326414279478e-12 -12.0249439982196 -78.9834959733178;-2e-06 -8.81214623374715e-12 -11.995167067934 -78.9880236576393;-1e-06 -8.81102707229702e-12 -11.9653884328676 -78.992540116001]  x5=2.03919101606495e-05  V1=ones(3,3)  V2=ones(3,3)  I1=ones(3,3)  I2=ones(3,3)  nHarmo=1  Measurements=None
  Ground3 : powerlib/Elements/Ground  LConnTagsString=a
  "Grounding Transformer " : powerlib/Elements/Grounding Transformer   UNITS=pu  NominalPower="[100e6   60]"  NominalVoltage=25e3  ZeroSequenceImpedance_pu=[0.025 0.75]  MagnetizationBranch_pu=[500 500]  ZeroSequenceImpedance_SI=[0.052083 589.05]  MagnetizationBranch_SI=[1041.7 3.927e+005]  Measurements=None
  A : PMIOPort  Port=1  Side=Left
  B : PMIOPort  Port=2  Side=Left
  C : PMIOPort  Port=3  Side=Left
  connections:
  "3.3ohms "/RConn1 -- Ground3/LConn1
  120 kV / 25 kV 47 MVA/LConn1 -- 120kV 2500MVA/RConn1
  120 kV / 25 kV 47 MVA/LConn2 -- 120kV 2500MVA/RConn2
  120 kV / 25 kV 47 MVA/LConn3 -- 120kV 2500MVA/RConn3
  120 kV / 25 kV 47 MVA/RConn1 -- "Grounding Transformer "/LConn1 -- 14-km Feeder/RConn1 -- 30-MW 2-Mvar Load/LConn1
  120 kV / 25 kV 47 MVA/RConn2 -- "Grounding Transformer "/LConn2 -- 14-km Feeder/RConn2 -- 30-MW 2-Mvar Load/LConn2
  120 kV / 25 kV 47 MVA/RConn3 -- "Grounding Transformer "/LConn3 -- 14-km Feeder/RConn3 -- 30-MW 2-Mvar Load/LConn3
  5-km Feeder/RConn1 -- 14-km Feeder/LConn1 -- 2-MW Load/LConn1
  5-km Feeder/RConn2 -- 14-km Feeder/LConn2 -- 2-MW Load/LConn2
  5-km Feeder/RConn3 -- 14-km Feeder/LConn3 -- 2-MW Load/LConn3
  A/RConn1 -- 5-km Feeder/LConn1
  B/RConn1 -- 5-km Feeder/LConn2
  C/RConn1 -- 5-km Feeder/LConn3
  "Grounding Transformer "/RConn1 -- "3.3ohms "/LConn1

== system power_PVarray_grid_det/Irradiance Temp ==
  Demux : Demux  Tag=STV Demux  Outputs=2
  FromWs : FromWorkspace  Tag=STV FromWs  VariableName=tuvar  SampleTime=0  SigBuilderData=DataTag0  VnvData=DataTag1
      SigBuilderData=|
      | common.afterFinalStr = 'Extrapolate'
      | common.sampleTime = '0'
      | dataSet(1).timeRange = [0 2]
      | dataSet(1).name = 'Constant Irradiance'
      | dataSet(2).timeRange = [0 2]
      | dataSet(2).name = 'Step Irradiance'
      | dataSet(3).timeRange = [0 3]
      | dataSet(3).name = 'Ramp-up/down Irradiance'
      | sbobj.Groups(1).Name = 'Constant Irradiance'
      | sbobj.Groups(1).Signals(1).Name = 'Ir'
      | sbobj.Groups(1).Signals(1).XData = [0 2]
      | sbobj.Groups(1).Signals(1).YData = [1000 1000]
      | sbobj.Groups(1).Signals(2).Name = 'Temp'
      | sbobj.Groups(1).Signals(2).XData = [0 1 1 2]
      | sbobj.Groups(1).Signals(2).YData = [0 0 1 1]
      | sbobj.Groups(1).TimeRange = [0 2]
      | sbobj.Groups(2).Name = 'Step Irradiance'
      | sbobj.Groups(2).Signals(1).Name = 'Ir'
      | sbobj.Groups(2).Signals(1).XData = [0 0.252 0.252 2]
      | sbobj.Groups(2).Signals(1).YData = [600 600 1000 1000]
      | sbobj.Groups(2).Signals(2).Name = 'Temp'
      | sbobj.Groups(2).Signals(2).XData = [0 1 1 2]
      | sbobj.Groups(2).Signals(2).YData = [0 0 1 1]
      | sbobj.Groups(2).TimeRange = [0 2]
      | sbobj.Groups(3).Name = 'Ramp-up/down Irradiance'
      | sbobj.Groups(3).Signals(1).Name = 'Ir'
      | sbobj.Groups(3).Signals(1).XData = [0 0.6 1.1 1.2 1.7 3]
      | sbobj.Groups(3).Signals(1).YData = [1000 1000 250 250 1000 1000]
      | sbobj.Groups(3).Signals(2).Name = 'Temp'
      | sbobj.Groups(3).Signals(2).XData = [0 2 2.1 3]
      | sbobj.Groups(3).Signals(2).YData = [25 25 50 50]
      | sbobj.Groups(3).TimeRange = [0 3]
  Ir : Outport  Tag=STV Outport
  Temp : Outport  Tag=STV Outport  Port=2
  wires:
  FromWs/1 -> Demux/1
  Demux/1 -> Ir/1
  Demux/2 -> Temp/1

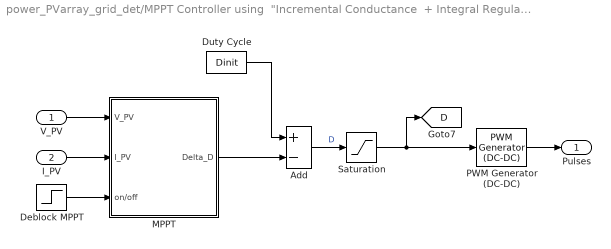
== system power_PVarray_grid_det/MPPT Controller using  "Incremental Conductance  + Integral Regulator "  technique  ==
  V_PV : Inport
  I_PV : Inport  Port=2
  Add : Sum  Inputs=+-
  Deblock MPPT : Step  Time=0.4  SampleTime=0
  Duty Cycle : Constant  Value=Dinit
  MPPT : Subsystem
  PWM Generator (DC-DC) : powerlib_meascontrol/Pulse & Signal Generators/PWM Generator (DC-DC)  Fsw=fc  Ts=Ts_Power
  Saturation : Saturate  UpperLimit=1  LowerLimit=0
  Pulses : Outport
  tag scope: D=global
  wires:
  V_PV/1 -> MPPT/1(V_PV)
  I_PV/1 -> MPPT/2(I_PV)
  PWM Generator (DC-DC)/1 -> Pulses/1
  Deblock MPPT/1 -> MPPT/3(on/off)
  Saturation/1 -> PWM Generator (DC-DC)/1, [D]
  Add/1 -> Saturation/1  "D"
  MPPT/1(Delta_D) -> Add/2
  Duty Cycle/1 -> Add/1

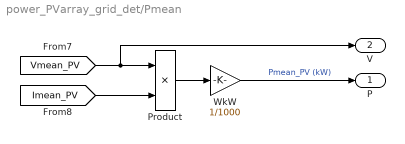
== system power_PVarray_grid_det/Pmean ==
  Product : Product  RndMeth=Zero
  WkW : Gain  Gain=1/1000
  P : Outport
  V : Outport  Port=2
  wires:
  [Vmean_PV] -> Product/1, V/1
  Product/1 -> WkW/1
  [Imean_PV] -> Product/2
  WkW/1 -> P/1  "Pmean_PV (kW)"

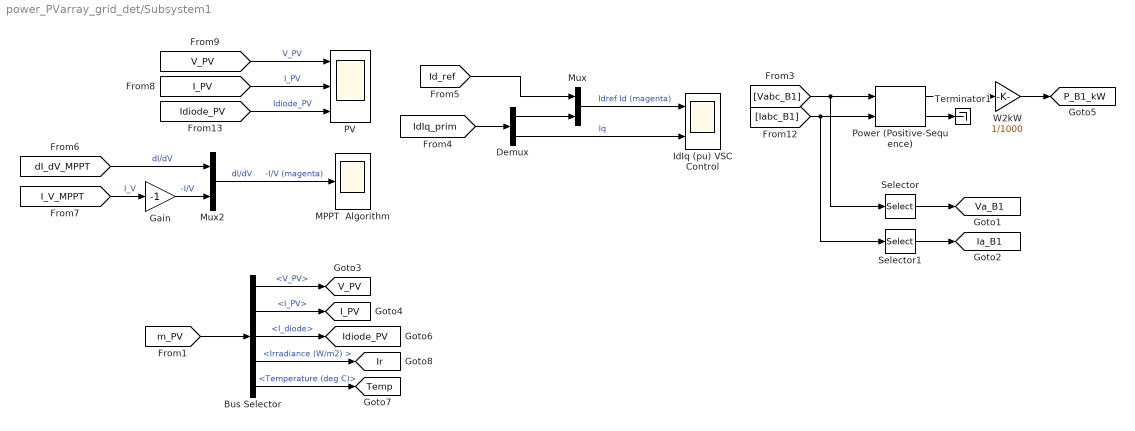
== system power_PVarray_grid_det/Subsystem1 ==
  Bus Selector : BusSelector  OutputSignals=V_PV,I_PV,I_diode,Irradiance (W/m2) ,Temperature (deg C)
  Demux : Demux  Outputs=2
  Gain : Gain  Gain=-1
  IdIq (pu) VSC Control : Scope  NumInputPorts=2
  MPPT  Algorithm : Scope
  Mux : Mux  Inputs=2
  Mux2 : Mux  Inputs=2
  PV : Scope  NumInputPorts=3
  Power (Positive-Sequence) : powerlib_meascontrol/Measurements/Power (Positive-Sequence)  Freq=60  Vinit=[0, 0]  Iinit=[0, 0]  Ts=Ts_Control
  Selector : Selector  InputPortWidth=3  IndexOptions=Index vector (dialog)  Indices=[1]  OutputSizes=1
  Selector1 : Selector  InputPortWidth=3  IndexOptions=Index vector (dialog)  Indices=[1]  OutputSizes=1
  Terminator1 : Terminator
  W2kW : Gain  Gain=1/1000
  tag scope: I_PV=global, Ia_B1=global, Idiode_PV=global, Ir=global, P_B1_kW=global, Temp=global, V_PV=global, Va_B1=global
  wires:
  [Vabc_B1] -> Power (Positive-Sequence)/1, Selector/1
  [Iabc_B1] -> Power (Positive-Sequence)/2, Selector1/1
  Power (Positive-Sequence)/1 -> W2kW/1
  [I_V_MPPT] -> Gain/1  "I_V"
  [IdIq_prim] -> Demux/1
  [Id_ref] -> Mux/1
  Demux/1 -> Mux/2
  Mux/1 -> IdIq (pu) VSC Control/1  "Idref Id (magenta)"
  Demux/2 -> IdIq (pu) VSC Control/2  "Iq"
  Selector/1 -> [Va_B1]
  Selector1/1 -> [Ia_B1]
  [V_PV] -> PV/1  "V_PV"
  [I_PV] -> PV/2  "I_PV"
  [Idiode_PV] -> PV/3  "Idiode_PV"
  [dI_dV_MPPT] -> Mux2/1  "dI/dV"
  Gain/1 -> Mux2/2  "-I/V"
  Mux2/1 -> MPPT  Algorithm/1  "dI/dV     -I/V (magenta)"
  W2kW/1 -> [P_B1_kW]
  [m_PV] -> Bus Selector/1
  Bus Selector/1 -> [V_PV]  "<V_PV>"
  Bus Selector/2 -> [I_PV]  "<I_PV>"
  Bus Selector/4 -> [Ir]  "<Irradiance (W/m2) >"
  Bus Selector/3 -> [Idiode_PV]  "<I_diode>"
  Bus Selector/5 -> [Temp]  "<Temperature (deg C)>"
  Power (Positive-Sequence)/2 -> Terminator1/1

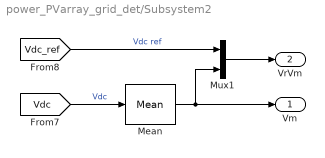
== system power_PVarray_grid_det/Subsystem2 ==
  Mean : powerlib_meascontrol/Measurements/Mean  Freq=60  Vinit=0  Ts=Ts_Control
  Mux1 : Mux  Inputs=2
  Vm : Outport
  VrVm : Outport  Port=2
  wires:
  [Vdc_ref] -> Mux1/1  "Vdc ref"
  [Vdc] -> Mean/1  "Vdc"
  Mux1/1 -> VrVm/1
  Mean/1 -> Mux1/2, Vm/1

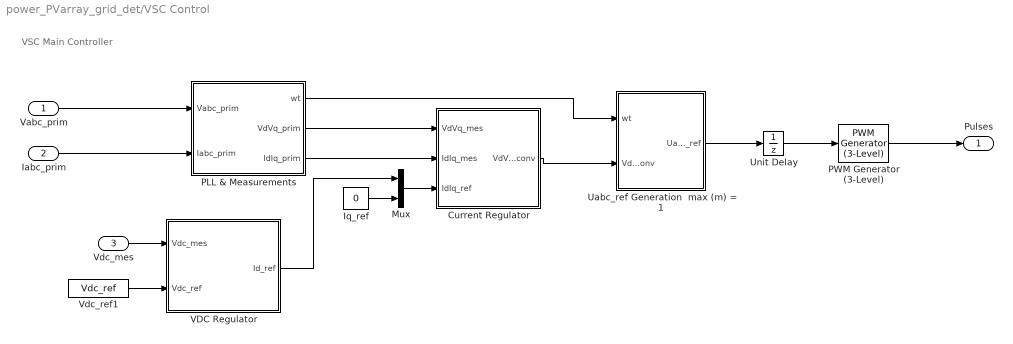
== system power_PVarray_grid_det/VSC Control ==
  note: VSC Main Controller
  Vabc_prim : Inport  PortDimensions=3
  Iabc_prim : Inport  Port=2  PortDimensions=3
  Vdc_mes : Inport  Port=3  PortDimensions=1
  Current Regulator : Subsystem
  Iq_ref : Constant  Value=0
  Mux : Mux  Inputs=2
  PLL & Measurements : Subsystem
  PWM Generator (3-Level) : powerlib_meascontrol/Pulse & Signal Generators/PWM Generator (3-Level)  ModulatorType=Three-phase bridge (12 pulses)  ModulatorMode=Unsynchronized  nF=27  Fc=33*60  ModulatingSignals=off  m=0.8  Freq=60  Phase=0  Ts=Ts_Power
  Uabc_ref Generation  max (m) = 1 : Subsystem
  Unit Delay : UnitDelay  SampleTime=Ts_Control
  VDC Regulator : Subsystem
  Vdc_ref1 : Constant  Value=Vdc_ref
  Pulses : Outport
  wires:
  VDC Regulator/1(Id_ref) -> Mux/1
  PLL & Measurements/1(wt) -> Uabc_ref Generation  max (m) = 1/1(wt)
  Current Regulator/1(VdVq_conv) -> Uabc_ref Generation  max (m) = 1/2(VdVq_conv)
  Iq_ref/1 -> Mux/2
  Mux/1 -> Current Regulator/3(IdIq_ref)
  PLL & Measurements/3(IdIq_prim) -> Current Regulator/2(IdIq_mes)
  PLL & Measurements/2(VdVq_prim) -> Current Regulator/1(VdVq_mes)
  Vdc_mes/1 -> VDC Regulator/1(Vdc_mes)
  Vabc_prim/1 -> PLL & Measurements/1(Vabc_prim)
  Iabc_prim/1 -> PLL & Measurements/2(Iabc_prim)
  Unit Delay/1 -> PWM Generator (3-Level)/1
  PWM Generator (3-Level)/1 -> Pulses/1
  Uabc_ref Generation  max (m) = 1/1(Uabc_ref) -> Unit Delay/1
  Vdc_ref1/1 -> VDC Regulator/2(Vdc_ref)

== system power_PVarray_grid_det/info ==

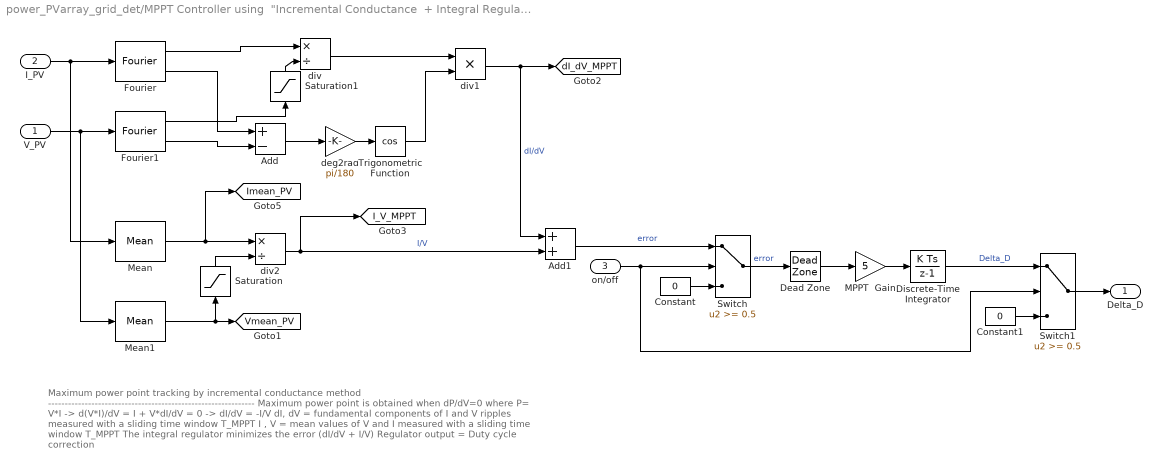
== system power_PVarray_grid_det/MPPT Controller using  "Incremental Conductance  + Integral Regulator "  technique /MPPT ==
  note: Maximum power point tracking by incremental conductance method
      | --------------------------------------------------------------
      | Maximum power point is obtained when dP/dV=0  where P= V*I
      | -> d(V*I)/dV = I + V*dI/dV = 0
      | -> dI/dV = -I/V
      |
      | dI, dV  = fundamental components of I and V ripples measured with a sliding time window T_MPPT
      | I , V   = mean values of V and I measured with a sliding time window T_MPPT
      |
      | The integral regulator minimizes the error (dI/dV + I/V)
      | Regulator output = Duty cycle correction
  V_PV : Inport
  I_PV : Inport  Port=2
  on/off : Inport  Port=3
  Add : Sum  Inputs=+-
  Add1 : Sum
  Constant : Constant  Value=0
  Constant1 : Constant  Value=0
  Dead Zone : DeadZone  LowerValue=-0.05  UpperValue=0.05  SaturateOnIntegerOverflow=on
  Discrete-Time Integrator : DiscreteIntegrator  SampleTime=Ts_Control  LimitOutput=on  UpperSaturationLimit=1  LowerSaturationLimit=-1  ICPrevOutput=DiscIntNeverNeededParam  ICPrevScaledInput=DiscIntNeverNeededParam
  Fourier : powerlib_meascontrol/Measurements/Fourier  Freq=1/T_MPPT  n=1  InInit=[0, 0]  Ts=Ts_Control
  Fourier1 : powerlib_meascontrol/Measurements/Fourier  Freq=1/T_MPPT  n=1  InInit=[0, 0]  Ts=Ts_Control
  MPPT  Gain : Gain  Gain=5
  Mean : powerlib_meascontrol/Measurements/Mean  Freq=1/T_MPPT  Vinit=0  Ts=Ts_Control
  Mean1 : powerlib_meascontrol/Measurements/Mean  Freq=1/T_MPPT  Vinit=0  Ts=Ts_Control
  Saturation : Saturate  UpperLimit=inf  LowerLimit=eps
  Saturation1 : Saturate  UpperLimit=inf  LowerLimit=eps
  Switch : Switch  Threshold=0.5
  Switch1 : Switch  Threshold=0.5
  Trigonometric Function : Trigonometry  Operator=cos
  deg2rad : Gain  Gain=pi/180
  div : Product  Inputs=*/  RndMeth=Zero
  div1 : Product  Inputs=**  RndMeth=Zero
  div2 : Product  Inputs=*/  RndMeth=Zero
  Delta_D : Outport
  tag scope: I_V_MPPT=global, Imean_PV=global, Vmean_PV=global, dI_dV_MPPT=global
  wires:
  Dead Zone/1 -> MPPT  Gain/1
  Switch/1 -> Dead Zone/1  "error"
  Saturation1/1 -> div/2
  Saturation/1 -> div2/2
  Switch1/1 -> Delta_D/1
  on/off/1 -> Switch/2, Switch1/2
  Constant1/1 -> Switch1/3
  Discrete-Time Integrator/1 -> Switch1/1  "Delta_D"
  Constant/1 -> Switch/3
  MPPT  Gain/1 -> Discrete-Time Integrator/1
  Add1/1 -> Switch/1  "error"
  div2/1 -> Add1/2, [I_V_MPPT]  "I/V"
  Mean1/1 -> Saturation/1, [Vmean_PV]
  Mean/1 -> div2/1, [Imean_PV]
  div1/1 -> Add1/1, [dI_dV_MPPT]  "dI/dV"
  Trigonometric Function/1 -> div1/2
  div/1 -> div1/1
  deg2rad/1 -> Trigonometric Function/1
  Add/1 -> deg2rad/1
  Fourier1/1 -> Saturation1/1
  Fourier1/2 -> Add/2
  Fourier/2 -> Add/1
  V_PV/1 -> Mean1/1, Fourier1/1
  I_PV/1 -> Mean/1, Fourier/1
  Fourier/1 -> div/1

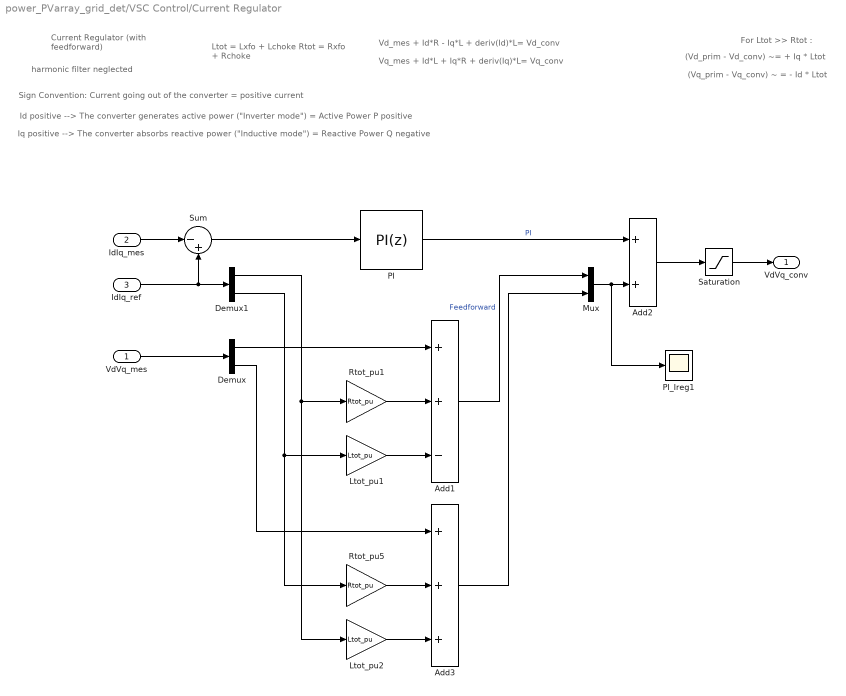
== system power_PVarray_grid_det/VSC Control/Current Regulator ==
  note: harmonic filter neglected
  note: Vd_mes + Id*R - Iq*L + deriv(Id)*L= Vd_conv
  note: Vq_mes + Id*L + Iq*R + deriv(Iq)*L= Vq_conv
  note: Current Regulator
      | (with feedforward)
  note: Sign Convention: Current going out of the converter = positive current
  note: Iq positive --> The converter absorbs reactive power ("Inductive mode") = Reactive Power Q negative
  note: Id positive --> The converter generates active power ("Inverter mode") = Active Power P positive
  note: Ltot = Lxfo + Lchoke
      | Rtot = Rxfo + Rchoke
  note: (Vd_prim - Vd_conv) ~= + Iq * Ltot
  note: (Vq_prim - Vq_conv) ~ = - Id * Ltot
  note: For Ltot >> Rtot :
  VdVq_mes : Inport  PortDimensions=2
  IdIq_mes : Inport  Port=2  PortDimensions=2
  IdIq_ref : Inport  Port=3  PortDimensions=2
  Add1 : Sum  Inputs=++-
  Add2 : Sum
  Add3 : Sum  Inputs=+++
  Demux : Demux  Outputs=2
  Demux1 : Demux  Outputs=2
  Ltot_pu1 : Gain  Gain=Ltot_pu  SaturateOnIntegerOverflow=on  OutDataTypeStr=Inherit: Same as input  ParamDataTypeStr=Inherit: Same as input
  Ltot_pu2 : Gain  Gain=Ltot_pu  SaturateOnIntegerOverflow=on  OutDataTypeStr=Inherit: Same as input  ParamDataTypeStr=Inherit: Same as input
  Mux : Mux  Inputs=2
  PI : simulink/Continuous/PID Controller  Controller=PI  TimeDomain=Discrete-time  SampleTime=Ts  IntegratorMethod=Forward Euler  FilterMethod=Forward Euler  Form=Parallel  UseFilter=on  ControllerParametersSource=internal  P=Kp_Ireg  I=Ki_Ireg  D=0  N=100  InitialConditionSource=internal  InitialConditionForIntegrator=0  InitialConditionForFilter=0  ExternalReset=none  LimitOutput=on  UpperSaturationLimit=2  LowerSaturationLimit=-2  LinearizeAsGain=off  AntiWindupMode=none  Kb=1  TrackingMode=off  Kt=1  PParamMin=[]  PParamMax=[]  IParamMin=[]  IParamMax=[]  DParamMin=[]  DParamMax=[]  NParamMin=[]  NParamMax=[]  KbParamMin=[]  KbParamMax=[]  KtParamMin=[]  KtParamMax=[]  POutMin=[]  POutMax=[]  IOutMin=[]  IOutMax=[]  DOutMin=[]  DOutMax=[]  NOutMin=[]  NOutMax=[]  KbOutMin=[]  KbOutMax=[]  KtOutMin=[]  KtOutMax=[]  IntegratorOutMin=[]  IntegratorOutMax=[]  FilterOutMin=[]  FilterOutMax=[]  SumOutMin=[]  SumOutMax=[]  SumI1OutMin=[]  SumI1OutMax=[]  SumI2OutMin=[]  SumI2OutMax=[]  SumI3OutMin=[]  SumI3OutMax=[]  SumDOutMin=[]  SumDOutMax=[]  SaturationOutMin=[]  SaturationOutMax=[]  IntegratorContinuousStateAttributes=''  IntegratorStateMustResolveToSignalObject=off  IntegratorRTWStateStorageClass=Auto  FilterContinuousStateAttributes=''  FilterStateMustResolveToSignalObject=off  FilterRTWStateStorageClass=Auto  DifferentiatorICPrevScaledInput=0  DifferentiatorOutMin=[]  DifferentiatorOutMax=[]
  PI_Ireg1 : Scope
  Rtot_pu1 : Gain  Gain=Rtot_pu  SaturateOnIntegerOverflow=on  OutDataTypeStr=Inherit: Same as input  ParamDataTypeStr=Inherit: Same as input
  Rtot_pu5 : Gain  Gain=Rtot_pu  SaturateOnIntegerOverflow=on  OutDataTypeStr=Inherit: Same as input  ParamDataTypeStr=Inherit: Same as input
  Saturation : Saturate  UpperLimit=2  LowerLimit=-2
  Sum : Sum  Inputs=|-+
  VdVq_conv : Outport
  wires:
  Mux/1 -> PI_Ireg1/1, Add2/2
  PI/1 -> Add2/1  "PI"
  Sum/1 -> PI/1
  IdIq_ref/1 -> Sum/2, Demux1/1
  IdIq_mes/1 -> Sum/1
  Add2/1 -> Saturation/1
  Saturation/1 -> VdVq_conv/1
  VdVq_mes/1 -> Demux/1
  Demux/1 -> Add1/1
  Rtot_pu1/1 -> Add1/2
  Demux1/1 -> Rtot_pu1/1, Ltot_pu2/1
  Ltot_pu1/1 -> Add1/3
  Demux1/2 -> Ltot_pu1/1, Rtot_pu5/1
  Rtot_pu5/1 -> Add3/2
  Ltot_pu2/1 -> Add3/3
  Add1/1 -> Mux/1  "Feedforward"
  Demux/2 -> Add3/1
  Add3/1 -> Mux/2

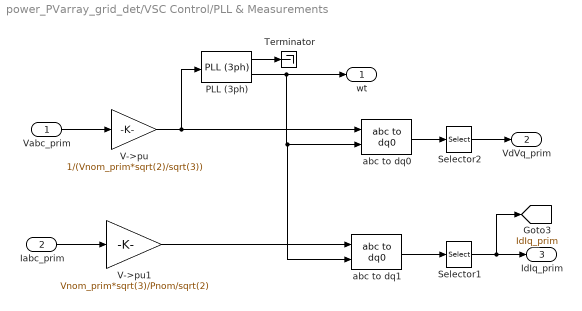
== system power_PVarray_grid_det/VSC Control/PLL & Measurements ==
  Vabc_prim : Inport
  Iabc_prim : Inport  Port=2
  PLL (3ph) : powerlib_meascontrol/PLL/PLL (3ph)  Fmin=45  Par_Init="[-0.57  Fnom]"  ParK=[180, 3200, 1]  TcD=1e-4  MaxRateChangeFreq=12  FilterCutOffFreq=25  Ts=Ts  AGC=on
  Selector1 : Selector  InputPortWidth=3  IndexOptions=Index vector (dialog)  Indices=[1 2]  OutputSizes=1
  Selector2 : Selector  InputPortWidth=3  IndexOptions=Index vector (dialog)  Indices=[1 2]  OutputSizes=1
  Terminator : Terminator
  V->pu : Gain  Gain=1/(Vnom_prim*sqrt(2)/sqrt(3))  SaturateOnIntegerOverflow=on  OutDataTypeStr=Inherit: Same as input  ParamDataTypeStr=Inherit: Same as input
  V->pu1 : Gain  Gain=Vnom_prim*sqrt(3)/Pnom/sqrt(2)  SaturateOnIntegerOverflow=on  OutDataTypeStr=Inherit: Same as input  ParamDataTypeStr=Inherit: Same as input
  abc to dq0 : powerlib_meascontrol/Transformations/abc to dq0  Alignment=90 degrees behind phase A axis
  abc to dq1 : powerlib_meascontrol/Transformations/abc to dq0  Alignment=90 degrees behind phase A axis
  wt : Outport
  VdVq_prim : Outport  Port=2
  IdIq_prim : Outport  Port=3
  tag scope: IdIq_prim=global
  wires:
  V->pu1/1 -> abc to dq1/1
  V->pu/1 -> PLL (3ph)/1, abc to dq0/1
  abc to dq1/1 -> Selector1/1
  Vabc_prim/1 -> V->pu/1
  Iabc_prim/1 -> V->pu1/1
  abc to dq0/1 -> Selector2/1
  Selector2/1 -> VdVq_prim/1
  Selector1/1 -> [IdIq_prim], IdIq_prim/1
  PLL (3ph)/2 -> wt/1, abc to dq1/2, abc to dq0/2
  PLL (3ph)/1 -> Terminator/1

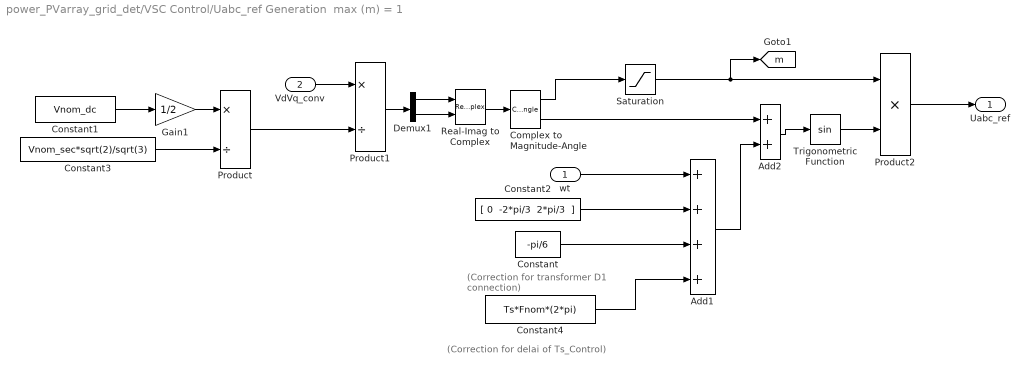
== system power_PVarray_grid_det/VSC Control/Uabc_ref Generation  max (m) = 1 ==
  note: (Correction for transformer
      |  D1 connection)
  note: (Correction for delai of Ts_Control)
  wt : Inport
  VdVq_conv : Inport  Port=2
  Add1 : Sum  Inputs=++++
  Add2 : Sum
  Complex to Magnitude-Angle : ComplexToMagnitudeAngle
  Constant : Constant  Value=-pi/6
  Constant1 : Constant  Value=Vnom_dc
  Constant2 : Constant  Value="[ 0  -2*pi/3  2*pi/3  ]"
  Constant3 : Constant  Value=Vnom_sec*sqrt(2)/sqrt(3)
  Constant4 : Constant  Value=Ts*Fnom*(2*pi)
  Demux1 : Demux  Outputs=2
  Gain1 : Gain  Gain=1/2
  Product : Product  Inputs=*/  RndMeth=Zero
  Product1 : Product  Inputs=*/  RndMeth=Zero
  Product2 : Product  Inputs=**  RndMeth=Zero
  Real-Imag to Complex : RealImagToComplex
  Saturation : Saturate  UpperLimit=1  LowerLimit=0
  Trigonometric Function : Trigonometry
  Uabc_ref : Outport
  tag scope: m=global
  wires:
  Complex to Magnitude-Angle/1 -> Saturation/1
  Constant1/1 -> Gain1/1
  VdVq_conv/1 -> Product1/1
  Product1/1 -> Demux1/1
  Gain1/1 -> Product/1
  Real-Imag to Complex/1 -> Complex to Magnitude-Angle/1
  Demux1/1 -> Real-Imag to Complex/1
  Demux1/2 -> Real-Imag to Complex/2
  Constant2/1 -> Add1/2
  Constant/1 -> Add1/3
  Constant3/1 -> Product/2
  Product/1 -> Product1/2
  Complex to Magnitude-Angle/2 -> Add2/1
  Add1/1 -> Add2/2
  Add2/1 -> Trigonometric Function/1
  Saturation/1 -> [m], Product2/1
  Trigonometric Function/1 -> Product2/2
  Product2/1 -> Uabc_ref/1
  wt/1 -> Add1/1
  Constant4/1 -> Add1/4
